simulink model "slosh_separated_with_controller"  (R2025b)
settings: Solver=ode45  StartTime=0.0  StopTime=20  RelTol=1e-3
libraries: slpidlib x1
settings Model: Creator=piepe  LastModifiedBy=piepe

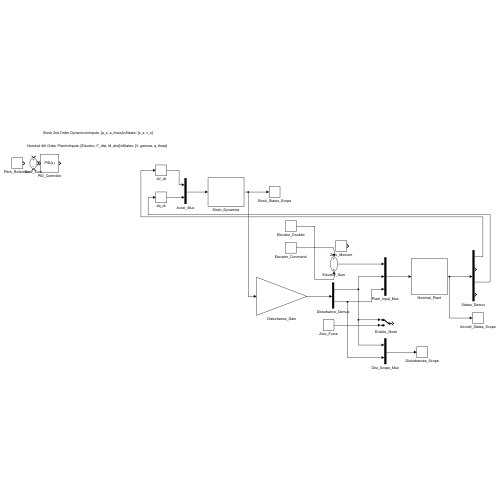
[thumbnail: Simulink's stored preview of the top-level diagram]
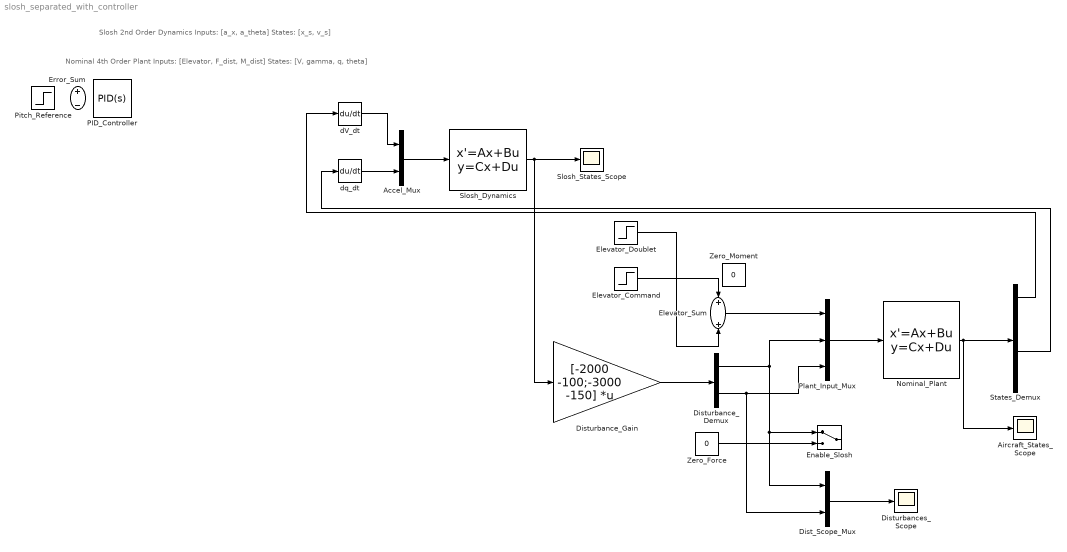
== system slosh_separated_with_controller ==
  note: Nominal 4th Order Plant\nInputs: [Elevator, F_dist, M_dist]\nStates: [V, gamma, q, theta]
  note: Slosh 2nd Order Dynamics\nInputs: [a_x, a_theta]\nStates: [x_s, v_s]
  Accel_Mux : Mux  Inputs=2
  Aircraft_States_Scope : Scope
  Dist_Scope_Mux : Mux  Inputs=2
  Disturbance_Demux : Demux  Outputs=2
  Disturbance_Gain : Gain  Gain=[-2000 -100;-3000 -150]  Multiplication=Matrix(K*u)
  Disturbances_Scope : Scope
  Elevator_Command : Step  Time=2  After=0.1  SampleTime=0
  Elevator_Doublet : Step  Time=3  After=-0.1  SampleTime=0
  Elevator_Sum : Sum
  Enable_Slosh : ManualSwitch
  Error_Sum : Sum  Inputs=+-
  Nominal_Plant : StateSpace  A=[-0.05 -9.81 0 0;-0.01 0 1 0;0 -0.000327 -0.000133333333333333 0;0 0 1 0]  B=[0.0002 0.0002 0;0 0 0;-0.000333333333333333 0 6.66666666666667e-05;0 0 0]  C=[1 0 0 0;0 1 0 0;0 0 1 0;0 0 0 1]  D=[0 0 0;0 0 0;0 0 0;0 0 0]  InitialCondition=[0;0.05;0;0.05]
  PID_Controller : slpidlib/PID Controller  Controller=PID  Form=Parallel  TimeDomain=Continuous-time  UseExternalTs=off  SampleTime=-1  IntegratorMethod=Forward Euler  FilterMethod=Forward Euler  ControllerParametersSource=internal  P=10  I=1  UseKiTs=off  D=2  UseExternalDerivativeSource=off  N=100  UseFilter=on  TunerSelectOption=Transfer Function Based (PID Tuner App)  InitialConditionSource=internal  InitialConditionForIntegrator=0  InitialConditionForFilter=0  DifferentiatorICPrevScaledInput=0  ExternalReset=none  TrackingMode=off  Kt=1  LimitOutput=off  SatLimitsSource=internal  UpperSaturationLimit=inf  LowerSaturationLimit=-inf  LinearizeAsGain=on  AntiWindupMode=none  Kb=1  LimitIntegrator=off  UpperIntegratorSaturationLimit=inf  LowerIntegratorSaturationLimit=-inf  POutMin=[]  POutMax=[]  IOutMin=[]  IOutMax=[]  DOutMin=[]  DOutMax=[]  NOutMin=[]  NOutMax=[]  SumOutMin=[]  SumOutMax=[]  SaturationOutMin=[]  SaturationOutMax=[]  PParamMin=[]  PParamMax=[]  IParamMin=[]  IParamMax=[]  DParamMin=[]  DParamMax=[]  NParamMin=[]  NParamMax=[]  KbParamMin=[]  KbParamMax=[]  KtParamMin=[]  KtParamMax=[]  KbOutMin=[]  KbOutMax=[]  KtOutMin=[]  KtOutMax=[]  IntegratorOutMin=[]  IntegratorOutMax=[]  FilterOutMin=[]  FilterOutMax=[]  SumI1OutMin=[]  SumI1OutMax=[]  SumI2OutMin=[]  SumI2OutMax=[]  SumI3OutMin=[]  SumI3OutMax=[]  SumI4OutMin=[]  SumI4OutMax=[]  SumDOutMin=[]  SumDOutMax=[]  DifferentiatorOutMin=[]  DifferentiatorOutMax=[]  FilterDiffOutCoefMin=[]  FilterDiffOutCoefMax=[]  ReciprocalOutMin=[]  ReciprocalOutMax=[]  SumDenOutMin=[]  SumDenOutMax=[]  SumNumOutMin=[]  SumNumOutMax=[]  DivideOutMin=[]  DivideOutMax=[]  UdiffTsProdOutMin=[]  UdiffTsProdOutMax=[]  NTsProdOutMin=[]  NTsProdOutMax=[]  UintegralTsProdOutMin=[]  UintegralTsProdOutMax=[]  UngainTsProdOutMin=[]  UngainTsProdOutMax=[]  ClampingZeroOutDataTypeStr=Inherit: Inherit via back propagation  ClampingZeroOutMin=[]  ClampingZeroOutMax=[]  FilterDenConstantOutDataTypeStr=Inherit: Inherit via back propagation  FilterDenConstantOutMin=[]  FilterDenConstantOutMax=[]  PCopyOutDataTypeStr=Inherit: Inherit via back propagation  PCopyOutMin=[]  PCopyOutMax=[]  NCopyOutDataTypeStr=Inherit: Inherit via back propagation  NCopyOutMin=[]  NCopyOutMax=[]  IntegratorContinuousStateAttributes=''  IntegratorStateMustResolveToSignalObject=off  IntegratorRTWStateStorageClass=Auto  FilterContinuousStateAttributes=''  FilterStateMustResolveToSignalObject=off  FilterRTWStateStorageClass=Auto  ParallelPVariant=InternalParameters  IdealPVariant=Disabled  IVariant=InternalParameters  DVariant=InternalParameters  IntegratorVariant=Continuous  SatVariant=Disabled  AWVariant=Passthrough  PCopyVariant=Disabled  TRVariant=Disabled  FdbkBlocksVariant=Forward  IdealPFdbkVariant=Disabled  SatFdbkVariant=Disabled  DerivativeFilterVariant=ContFilter  NVariant=InternalParameters  NCopyVariant=Disabled  FilterICVariant=InternalICsFilter  IntegratorICVariant=InternalICs  ExternalResetVariant=Disabled  TRSumVariant=Passthrough  SumFdbkVariant=Disabled  SumVariant=Sum_PID  TsampFilterVariant=InternalTs  TsampNgainVariant=Passthrough  TsampIntegralVariant=Disabled_SignalSpec  ExternalSaturationOutDataTypeStr=Inherit: Same as second input  DerivativeSourceVariant=ErrorSignal  PreIntVariant=InternalPreInt
  Pitch_Reference : Step  After=0.1  SampleTime=0
  Plant_Input_Mux : Mux  Inputs=3
  Slosh_Dynamics : StateSpace  A=[0 1;-4 -0.2]  B=[0 0;1 1.5]  C=[1 0;0 1]  D=[0 0;0 0]  InitialCondition=[0.1;0]
  Slosh_States_Scope : Scope
  States_Demux : Demux
  Zero_Force : Constant  Value=0
  Zero_Moment : Constant  Value=0
  dV_dt : Derivative
  dq_dt : Derivative
  wires:
  dq_dt/1 -> Accel_Mux/2
  dV_dt/1 -> Accel_Mux/1
  Disturbance_Gain/1 -> Disturbance_Demux/1
  Slosh_Dynamics/1 -> Disturbance_Gain/1, Slosh_States_Scope/1
  Accel_Mux/1 -> Slosh_Dynamics/1
  Elevator_Command/1 -> Elevator_Sum/1
  Elevator_Doublet/1 -> Elevator_Sum/2
  Elevator_Sum/1 -> Plant_Input_Mux/1
  Disturbance_Demux/1 -> Dist_Scope_Mux/1, Enable_Slosh/1, Plant_Input_Mux/2
  Plant_Input_Mux/1 -> Nominal_Plant/1
  Disturbance_Demux/2 -> Dist_Scope_Mux/2, Plant_Input_Mux/3
  Dist_Scope_Mux/1 -> Disturbances_Scope/1
  Zero_Force/1 -> Enable_Slosh/2
  States_Demux/1 -> dV_dt/1
  Nominal_Plant/1 -> States_Demux/1, Aircraft_States_Scope/1
  States_Demux/3 -> dq_dt/1
